simulink model "DigitalCircuit"  (R2024b)
settings: Solver=VariableStepAuto  StartTime=0.0  StopTime=10.0  RelTol=1e-3
libraries: simulink_extras x2
settings Model: Creator=keita  LastModifiedBy=keita

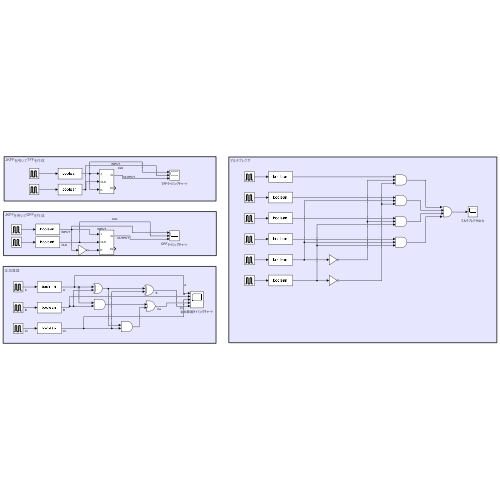
[thumbnail: Simulink's stored preview of the top-level diagram]
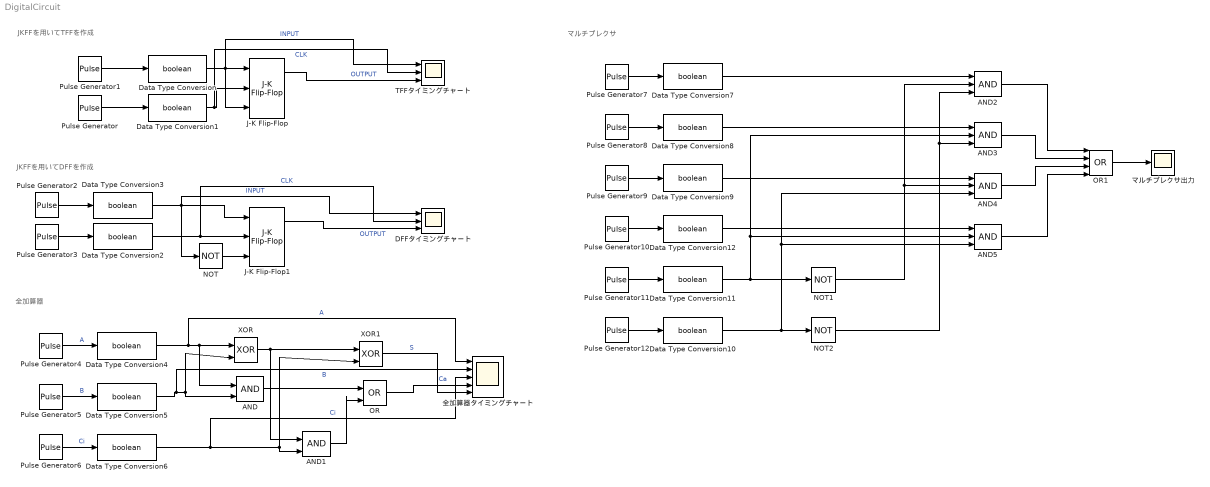
== system DigitalCircuit ==
  note: マルチプレクサ
  note: 全加算器
  note: JKFFを用いてTFFを作成
  note: JKFFを用いてDFFを作成
  AND : Logic  IconShape=distinctive  AllPortsSameDT=off  OutDataTypeStr=boolean
  AND1 : Logic  IconShape=distinctive  AllPortsSameDT=off  OutDataTypeStr=boolean
  AND{2..5} (4 alike) : Logic  Inputs=3  IconShape=distinctive  AllPortsSameDT=off  OutDataTypeStr=boolean
  DFFタイミングチャート : Scope  NumInputPorts=3
  Data Type Conversion{,1..12} (13 alike) : DataTypeConversion  OutDataTypeStr=boolean  SaturateOnIntegerOverflow=off  RndMeth=Floor
  J-K Flip-Flop : simulink_extras/Flip Flops/J-K Flip-Flop  initial_condition=0
  J-K Flip-Flop1 : simulink_extras/Flip Flops/J-K Flip-Flop  initial_condition=0
  NOT : Logic  Operator=NOT  IconShape=distinctive  AllPortsSameDT=off  OutDataTypeStr=boolean
  NOT1 : Logic  Operator=NOT  IconShape=distinctive  AllPortsSameDT=off  OutDataTypeStr=boolean
  NOT2 : Logic  Operator=NOT  IconShape=distinctive  AllPortsSameDT=off  OutDataTypeStr=boolean
  OR : Logic  Operator=OR  IconShape=distinctive  AllPortsSameDT=off  OutDataTypeStr=boolean
  OR1 : Logic  Operator=OR  Inputs=4  IconShape=distinctive  AllPortsSameDT=off  OutDataTypeStr=boolean
  Pulse Generator{,3,7..12} (8 alike) : DiscretePulseGenerator  PulseType=Time based  Period=1  PulseWidth=50
  Pulse Generator1 : DiscretePulseGenerator  PulseType=Time based  Period=4  PulseWidth=50
  Pulse Generator2 : DiscretePulseGenerator  PulseType=Time based  Period=4  PulseWidth=50
  Pulse Generator4 : DiscretePulseGenerator  PulseType=Time based  Period=10  PulseWidth=5
  Pulse Generator5 : DiscretePulseGenerator  PulseType=Time based  Period=10  PulseWidth=5
  Pulse Generator6 : DiscretePulseGenerator  PulseType=Time based  Period=10  PulseWidth=5
  TFFタイミングチャート : Scope  NumInputPorts=3
  XOR : Logic  Operator=XOR  IconShape=distinctive  AllPortsSameDT=off  OutDataTypeStr=boolean
  XOR1 : Logic  Operator=XOR  IconShape=distinctive  AllPortsSameDT=off  OutDataTypeStr=boolean
  マルチプレクサ出力 : Scope
  全加算器タイミングチャート : Scope  NumInputPorts=5
  wires:
  Pulse Generator1/1 -> Data Type Conversion/1
  Data Type Conversion/1 -> TFFタイミングチャート/1, J-K Flip-Flop/3, J-K Flip-Flop/1  "INPUT"
  Pulse Generator/1 -> Data Type Conversion1/1
  Data Type Conversion1/1 -> TFFタイミングチャート/2, J-K Flip-Flop/2  "CLK"
  J-K Flip-Flop/1 -> TFFタイミングチャート/3  "OUTPUT"
  Data Type Conversion2/1 -> DFFタイミングチャート/2, J-K Flip-Flop1/2  "CLK"
  Pulse Generator3/1 -> Data Type Conversion2/1
  Data Type Conversion3/1 -> DFFタイミングチャート/1, NOT/1, J-K Flip-Flop1/1  "INPUT"
  Pulse Generator2/1 -> Data Type Conversion3/1
  NOT/1 -> J-K Flip-Flop1/3
  J-K Flip-Flop1/1 -> DFFタイミングチャート/3  "OUTPUT"
  Data Type Conversion4/1 -> 全加算器タイミングチャート/1, XOR/1, AND/1  "A"
  Data Type Conversion5/1 -> 全加算器タイミングチャート/2, XOR/2, AND/2  "B"
  XOR/1 -> AND1/1, XOR1/1
  Data Type Conversion6/1 -> 全加算器タイミングチャート/3, XOR1/2, AND1/2  "Ci"
  AND/1 -> OR/1
  AND1/1 -> OR/2
  Pulse Generator4/1 -> Data Type Conversion4/1  "A"
  Pulse Generator5/1 -> Data Type Conversion5/1  "B"
  Pulse Generator6/1 -> Data Type Conversion6/1  "Ci"
  XOR1/1 -> 全加算器タイミングチャート/5  "S"
  OR/1 -> 全加算器タイミングチャート/4  "Ca"
  Data Type Conversion11/1 -> AND5/2, AND3/2, NOT1/1
  Data Type Conversion10/1 -> AND5/3, AND4/3, NOT2/1
  Data Type Conversion7/1 -> AND2/1
  Data Type Conversion8/1 -> AND3/1
  Data Type Conversion9/1 -> AND4/1
  Data Type Conversion12/1 -> AND5/1
  NOT1/1 -> AND4/2, AND2/2
  NOT2/1 -> AND3/3, AND2/3
  AND2/1 -> OR1/1
  AND3/1 -> OR1/2
  AND4/1 -> OR1/3
  AND5/1 -> OR1/4
  Pulse Generator7/1 -> Data Type Conversion7/1
  Pulse Generator8/1 -> Data Type Conversion8/1
  Pulse Generator9/1 -> Data Type Conversion9/1
  Pulse Generator10/1 -> Data Type Conversion12/1
  Pulse Generator11/1 -> Data Type Conversion11/1
  Pulse Generator12/1 -> Data Type Conversion10/1
  OR1/1 -> マルチプレクサ出力/1
